simulink model "gm_sampleModel2062_sub"  (R2023a)
settings: Solver=VariableStepAuto  StartTime=0.0  StopTime=10.0  RelTol=1e-3
libraries: simulink x2
settings Model: Creator=user1  LastModifiedBy=user1
settings OptimizationCC: BlockReduction=off  ConditionallyExecuteInputs=off
settings DebuggingCC: InheritedTsInSrcMsg=none

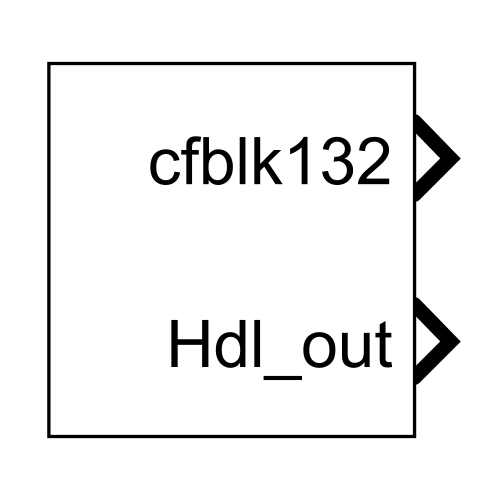
[thumbnail: Simulink's stored preview of the top-level diagram]
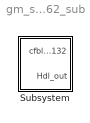
== system gm_sampleModel2062_sub ==
  Subsystem : Subsystem

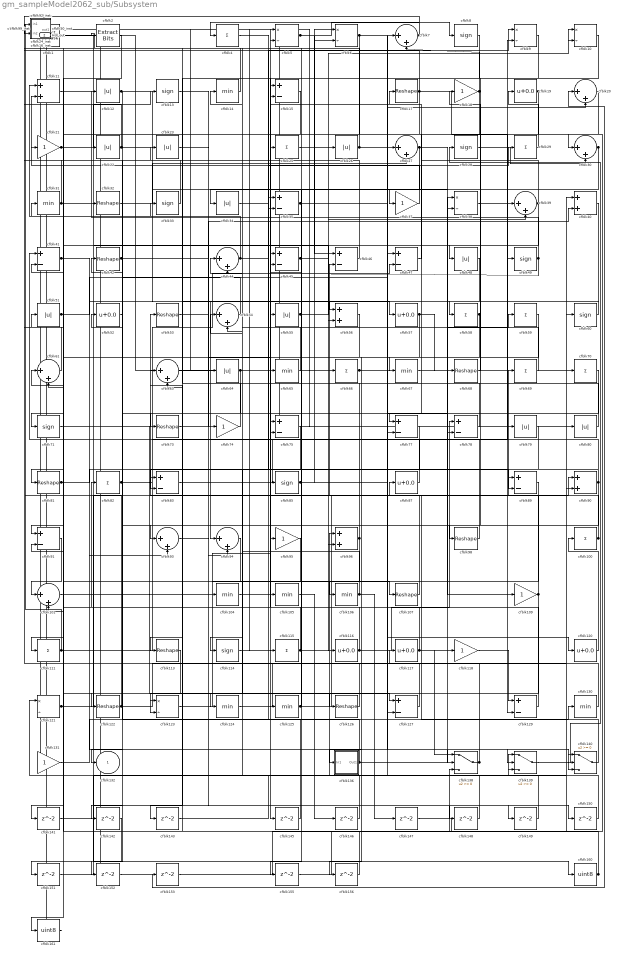
== system gm_sampleModel2062_sub/Subsystem ==
  cfblk1 : simulink/Logic and Bit Operations/Detect Decrease  vinit=0.0  OutDataTypeStr=uint8
      settings: LibrarySourceBlock=|
      | hdlsllib/Logic and Bit
      | Operations/Detect
      | Decrease
  cfblk{5..6,9..10,38,121,123} (7 alike) : Product  Inputs=*/  OutDataTypeStr=uint8  RndMeth=Zero  SaturateOnIntegerOverflow=on
  cfblk{4,25,29,58..59,66,69..70,82,100,111,115} (12 alike) : Sum  Inputs=+  OutDataTypeStr=uint8
  cfblk{7,20,27,30,39,44,54,61,63,93..94,101} (12 alike) : Sum  Inputs=|++  OutDataTypeStr=uint8
  cfblk{14,31,65,67,104..106,124..125,130} (10 alike) : MinMax  OutDataTypeStr=uint8
  cfblk{17,32,42,53,68,73,81,98,107,113,122,126} (12 alike) : Reshape
  cfblk108_inst : Subsystem
  cfblk{18,21,37,74,95,109,118,131} (8 alike) : Gain  OutDataTypeStr=uint8
  cfblk{11,40,56,90,96} (5 alike) : Sum  OutDataTypeStr=uint8
  cfblk112_inst : Subsystem
  cfblk{8,13,28,33,49,60,71,85,114} (9 alike) : Signum
  cfblk{19,52,57,87,116..117,120} (7 alike) : Bias  Bias=0.0  SaturateOnIntegerOverflow=off
  cfblk{12,22..23,26,34,48,51,55,64,79..80} (11 alike) : Abs  OutDataTypeStr=uint8  SaturateOnIntegerOverflow=off
  cfblk{15,35,41,45..47,75,77..78,83,89,91,127,129} (14 alike) : Sum  Inputs=+-  OutDataTypeStr=uint8
  cfblk136 : Subsystem
  cfblk138 : Switch  OutDataTypeStr=uint8  SaturateOnIntegerOverflow=off  InputSameDT=off
  cfblk139 : Switch  OutDataTypeStr=uint8  SaturateOnIntegerOverflow=off  InputSameDT=off
  cfblk140 : Switch  OutDataTypeStr=uint8  SaturateOnIntegerOverflow=off  InputSameDT=off
  cfblk{141..143,145..153,155..156} (14 alike) : Delay  SampleTime=1
  cfblk160 : DataTypeConversion  OutDataTypeStr=uint8  SaturateOnIntegerOverflow=off  RndMeth=Floor
  cfblk161 : DataTypeConversion  OutDataTypeStr=uint8  SaturateOnIntegerOverflow=off  RndMeth=Floor
  cfblk16_inst : Subsystem
  cfblk2 : simulink/Logic and Bit Operations/Extract Bits  bitsToExtract=Upper half  numBits=8  bitIdxRange=[0 7]  outScalingMode=Preserve fixed-point scaling
      settings: LibrarySourceBlock=|
      | hdlsllib/Logic and Bit
      | Operations/Extract Bits
  cfblk24_inst : Subsystem
  cfblk50_inst : Subsystem
  cfblk92_inst : Subsystem
  cfblk99_inst : Subsystem
  cfblk132 : Outport  OutDataTypeStr=uint8  SampleTime=1  VectorParamsAs1DForOutWhenUnconnected=off
  Hdl_out : Outport  Port=2  OutDataTypeStr=uint8  SampleTime=1
  wires:
  cfblk1/1 -> cfblk160/1
  cfblk10/1 -> cfblk145/1
  cfblk100/1 -> cfblk46/2, cfblk5/1
  cfblk101/1 -> cfblk107/1
  cfblk104/1 -> cfblk115/1
  cfblk105/1 -> cfblk146/1
  cfblk106/1 -> cfblk44/1, cfblk147/1
  cfblk107/1 -> cfblk53/1
  cfblk108_inst/1(out1) -> cfblk121/2
  cfblk109/1 -> cfblk123/2, cfblk14/1, cfblk69/1
  cfblk11/1 -> cfblk150/1
  cfblk111/1 -> cfblk47/2, cfblk24_inst/1(in1)
  cfblk112_inst/1(out1) -> cfblk131/1
  cfblk113/1 -> cfblk151/1
  cfblk114/1 -> cfblk9/1
  cfblk115/1 -> cfblk91/2, cfblk25/1
  cfblk116/1 -> cfblk92_inst/1(in1), cfblk78/1
  cfblk117/1 -> cfblk54/2, cfblk138/1, cfblk82/1
  cfblk118/1 -> cfblk129/1
  cfblk12/1 -> cfblk94/1, cfblk132/1
  cfblk120/1 -> cfblk100/1
  cfblk121/1 -> cfblk7/1, cfblk45/1, cfblk35/2
  cfblk122/1 -> cfblk92_inst/2(in2), cfblk117/1
  cfblk123/1 -> cfblk95/1
  cfblk124/1 -> cfblk60/1
  cfblk125/1 -> cfblk90/1, cfblk15/1
  cfblk126/1 -> cfblk52/1
  cfblk127/1 -> cfblk105/1
  cfblk129/1 -> cfblk5/2
  cfblk13/1 -> cfblk55/1
  cfblk130/1 -> cfblk61/1
  cfblk131/1 -> cfblk130/1
  cfblk136/1(Out1) -> cfblk42/1, cfblk38/1
  cfblk138/1 -> cfblk45/2, cfblk16_inst/1(in1)
  cfblk139/1 -> cfblk28/1
  cfblk14/1 -> cfblk2/1
  cfblk140/1 -> cfblk87/1
  cfblk141/1 -> cfblk40/1
  cfblk142/1 -> cfblk161/1
  cfblk143/1 -> cfblk139/1
  cfblk145/1 -> cfblk35/1
  cfblk146/1 -> cfblk54/1
  cfblk147/1 -> cfblk30/1
  cfblk148/1 -> cfblk96/1
  cfblk149/1 -> cfblk139/3
  cfblk15/1 -> cfblk101/2
  cfblk150/1 -> cfblk121/1
  cfblk151/1 -> cfblk27/1
  cfblk152/1 -> cfblk20/1
  cfblk153/1 -> cfblk138/3
  cfblk155/1 -> cfblk90/2
  cfblk156/1 -> cfblk41/2
  cfblk16_inst/1(out1) -> cfblk118/1
  cfblk160/1 -> cfblk63/1, cfblk51/1
  cfblk161/1 -> cfblk1/1
  cfblk17/1 -> cfblk81/1, cfblk50_inst/2(in2), cfblk129/2
  cfblk18/1 -> cfblk7/2, cfblk67/1
  cfblk19/1 -> cfblk93/1, cfblk63/2
  cfblk2/1 -> cfblk111/1
  cfblk20/1 -> cfblk98/1
  cfblk21/1 -> cfblk96/2, cfblk13/1
  cfblk22/1 -> cfblk108_inst/2(in2), cfblk38/2
  cfblk23/1 -> cfblk74/1
  cfblk24_inst/1(out1) -> cfblk79/1
  cfblk25/1 -> cfblk26/1
  cfblk26/1 -> cfblk140/3, cfblk120/1, cfblk112_inst/1(in1)
  cfblk27/1 -> cfblk155/1, cfblk109/1
  cfblk28/1 -> cfblk30/2
  cfblk29/1 -> cfblk19/1
  cfblk30/1 -> cfblk77/1, cfblk75/2, cfblk34/1
  cfblk31/1 -> cfblk16_inst/2(in2), cfblk116/1
  cfblk32/1 -> cfblk27/2
  cfblk33/1 -> cfblk99_inst/2(in2)
  cfblk34/1 -> cfblk37/1
  cfblk35/1 -> cfblk20/2, cfblk140/2
  cfblk37/1 -> cfblk11/2
  cfblk38/1 -> cfblk9/2
  cfblk39/1 -> cfblk71/1, cfblk15/2
  cfblk4/1 -> cfblk89/2
  cfblk40/1 -> cfblk125/1
  cfblk41/1 -> cfblk93/2, cfblk139/2
  cfblk42/1 -> cfblk56/1, cfblk65/1
  cfblk44/1 -> cfblk11/1, cfblk29/1
  cfblk45/1 -> cfblk56/2, cfblk6/2
  cfblk46/1 -> cfblk24_inst/2(in2)
  cfblk47/1 -> cfblk17/1
  cfblk48/1 -> cfblk143/1
  cfblk49/1 -> cfblk44/2, cfblk12/1
  cfblk5/1 -> cfblk8/1, cfblk46/1
  cfblk50_inst/1(out1) -> cfblk70/1
  cfblk51/1 -> cfblk57/1, cfblk47/1
  cfblk52/1 -> cfblk122/1
  cfblk53/1 -> cfblk94/2
  cfblk54/1 -> cfblk22/1
  cfblk55/1 -> cfblk39/2, cfblk10/1
  cfblk56/1 -> cfblk91/1
  cfblk57/1 -> cfblk75/1, cfblk68/1
  cfblk58/1 -> cfblk156/1, cfblk136/1(In1)
  cfblk59/1 -> cfblk64/1
  cfblk6/1 -> cfblk83/2, cfblk140/1
  cfblk60/1 -> cfblk58/1
  cfblk61/1 -> cfblk99_inst/1(in1)
  cfblk63/1 -> cfblk149/1
  cfblk64/1 -> cfblk73/1, Hdl_out/1
  cfblk65/1 -> cfblk108_inst/1(in1)
  cfblk66/1 -> cfblk78/2, cfblk10/2
  cfblk67/1 -> cfblk59/1
  cfblk68/1 -> cfblk18/1
  cfblk69/1 -> cfblk23/1
  cfblk7/1 -> cfblk112_inst/2(in2), cfblk4/1
  cfblk70/1 -> cfblk152/1
  cfblk71/1 -> cfblk127/1
  cfblk73/1 -> cfblk40/2
  cfblk74/1 -> cfblk33/1
  cfblk75/1 -> cfblk124/1
  cfblk77/1 -> cfblk126/1
  cfblk78/1 -> cfblk50_inst/1(in1)
  cfblk79/1 -> cfblk127/2
  cfblk8/1 -> cfblk113/1
  cfblk80/1 -> cfblk31/1
  cfblk81/1 -> cfblk89/1, cfblk138/2
  cfblk82/1 -> cfblk49/1, cfblk104/1
  cfblk83/1 -> cfblk39/1
  cfblk85/1 -> cfblk77/2, cfblk6/1
  cfblk87/1 -> cfblk61/2
  cfblk89/1 -> cfblk106/1
  cfblk9/1 -> cfblk48/1
  cfblk90/1 -> cfblk85/1, cfblk83/1, cfblk41/1, cfblk142/1
  cfblk91/1 -> cfblk101/1
  cfblk92_inst/1(out1) -> cfblk66/1
  cfblk93/1 -> cfblk148/1
  cfblk94/1 -> cfblk123/1
  cfblk95/1 -> cfblk141/1
  cfblk96/1 -> cfblk32/1, cfblk114/1
  cfblk98/1 -> cfblk21/1
  cfblk99_inst/1(out1) -> cfblk80/1, cfblk153/1

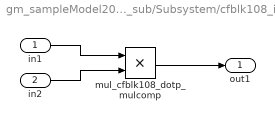
== system gm_sampleModel2062_sub/Subsystem/cfblk108_inst ==
  in1 : Inport  OutDataTypeStr=uint8  SampleTime=1
  in2 : Inport  Port=2  OutDataTypeStr=uint8  SampleTime=1
  mul_cfblk108_dotp_mulcomp : Product  Inputs=**  OutDataTypeStr=uint8  SampleTime=1
  out1 : Outport  OutDataTypeStr=uint8  SampleTime=1
  wires:
  in1/1 -> mul_cfblk108_dotp_mulcomp/1
  in2/1 -> mul_cfblk108_dotp_mulcomp/2
  mul_cfblk108_dotp_mulcomp/1 -> out1/1

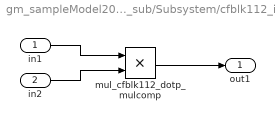
== system gm_sampleModel2062_sub/Subsystem/cfblk112_inst ==
  in1 : Inport  OutDataTypeStr=uint8  SampleTime=1
  in2 : Inport  Port=2  OutDataTypeStr=uint8  SampleTime=1
  mul_cfblk112_dotp_mulcomp : Product  Inputs=**  OutDataTypeStr=uint8  SampleTime=1
  out1 : Outport  OutDataTypeStr=uint8  SampleTime=1
  wires:
  in1/1 -> mul_cfblk112_dotp_mulcomp/1
  in2/1 -> mul_cfblk112_dotp_mulcomp/2
  mul_cfblk112_dotp_mulcomp/1 -> out1/1

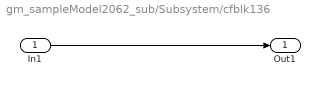
== system gm_sampleModel2062_sub/Subsystem/cfblk136 ==
  In1 : Inport  OutDataTypeStr=uint8  PortDimensions=1  SampleTime=1
  Out1 : Outport  SampleTime=1
  wires:
  In1/1 -> Out1/1

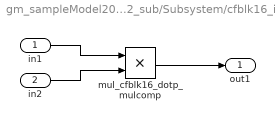
== system gm_sampleModel2062_sub/Subsystem/cfblk16_inst ==
  in1 : Inport  OutDataTypeStr=uint8  SampleTime=1
  in2 : Inport  Port=2  OutDataTypeStr=uint8  SampleTime=1
  mul_cfblk16_dotp_mulcomp : Product  Inputs=**  OutDataTypeStr=uint8  SampleTime=1
  out1 : Outport  OutDataTypeStr=uint8  SampleTime=1
  wires:
  in1/1 -> mul_cfblk16_dotp_mulcomp/1
  in2/1 -> mul_cfblk16_dotp_mulcomp/2
  mul_cfblk16_dotp_mulcomp/1 -> out1/1

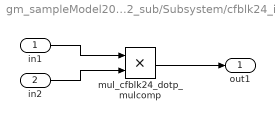
== system gm_sampleModel2062_sub/Subsystem/cfblk24_inst ==
  in1 : Inport  OutDataTypeStr=uint8  SampleTime=1
  in2 : Inport  Port=2  OutDataTypeStr=uint8  SampleTime=1
  mul_cfblk24_dotp_mulcomp : Product  Inputs=**  OutDataTypeStr=uint8  SampleTime=1
  out1 : Outport  OutDataTypeStr=uint8  SampleTime=1
  wires:
  in1/1 -> mul_cfblk24_dotp_mulcomp/1
  in2/1 -> mul_cfblk24_dotp_mulcomp/2
  mul_cfblk24_dotp_mulcomp/1 -> out1/1

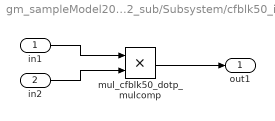
== system gm_sampleModel2062_sub/Subsystem/cfblk50_inst ==
  in1 : Inport  OutDataTypeStr=uint8  SampleTime=1
  in2 : Inport  Port=2  OutDataTypeStr=uint8  SampleTime=1
  mul_cfblk50_dotp_mulcomp : Product  Inputs=**  OutDataTypeStr=uint8  SampleTime=1
  out1 : Outport  OutDataTypeStr=uint8  SampleTime=1
  wires:
  in1/1 -> mul_cfblk50_dotp_mulcomp/1
  in2/1 -> mul_cfblk50_dotp_mulcomp/2
  mul_cfblk50_dotp_mulcomp/1 -> out1/1

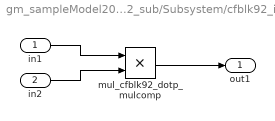
== system gm_sampleModel2062_sub/Subsystem/cfblk92_inst ==
  in1 : Inport  OutDataTypeStr=uint8  SampleTime=1
  in2 : Inport  Port=2  OutDataTypeStr=uint8  SampleTime=1
  mul_cfblk92_dotp_mulcomp : Product  Inputs=**  OutDataTypeStr=uint8  SampleTime=1
  out1 : Outport  OutDataTypeStr=uint8  SampleTime=1
  wires:
  in1/1 -> mul_cfblk92_dotp_mulcomp/1
  in2/1 -> mul_cfblk92_dotp_mulcomp/2
  mul_cfblk92_dotp_mulcomp/1 -> out1/1

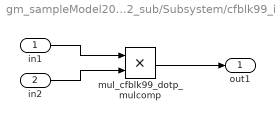
== system gm_sampleModel2062_sub/Subsystem/cfblk99_inst ==
  in1 : Inport  OutDataTypeStr=uint8  SampleTime=1
  in2 : Inport  Port=2  OutDataTypeStr=uint8  SampleTime=1
  mul_cfblk99_dotp_mulcomp : Product  Inputs=**  OutDataTypeStr=uint8  SampleTime=1
  out1 : Outport  OutDataTypeStr=uint8  SampleTime=1
  wires:
  in1/1 -> mul_cfblk99_dotp_mulcomp/1
  in2/1 -> mul_cfblk99_dotp_mulcomp/2
  mul_cfblk99_dotp_mulcomp/1 -> out1/1
